simulink model "SafetyChecks"  (R2020b)
settings: Solver=FixedStepDiscrete  StartTime=0.0  StopTime=10.0  FixedStep=4*Ts  RelTol=1e-3
undefined symbols (not defined in the file or in its folder): MaximumCurrentBeforeReaction
libraries: simulink x3
settings Model: DataDictionary=SafetyChecks.sldd  Creator=unix  LastModifiedBy=unix

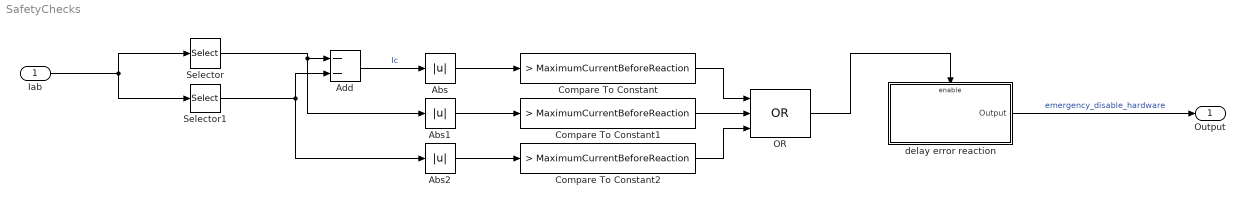
== system SafetyChecks ==
  Iab : Inport  OutDataTypeStr=fixdt(1,16,2^-8,0)
  Abs : Abs
  Abs1 : Abs
  Abs2 : Abs
  Add : Sum  Inputs=--
  Compare To Constant : simulink/Logic and Bit Operations/Compare To Constant  relop=>  const=MaximumCurrentBeforeReaction  OutDataTypeStr=boolean
  Compare To Constant1 : simulink/Logic and Bit Operations/Compare To Constant  relop=>  const=MaximumCurrentBeforeReaction  OutDataTypeStr=boolean
  Compare To Constant2 : simulink/Logic and Bit Operations/Compare To Constant  relop=>  const=MaximumCurrentBeforeReaction  OutDataTypeStr=boolean
  OR : Logic  Operator=OR  Inputs=3  IconShape=distinctive  AllPortsSameDT=off  OutDataTypeStr=boolean
  Selector : Selector  InputPortWidth=2  IndexOptions=Index vector (dialog)  Indices=[1]  OutputSizes=1
  Selector1 : Selector  InputPortWidth=2  IndexOptions=Index vector (dialog)  Indices=[2]  OutputSizes=1
  delay error reaction : Subsystem  TreatAsAtomicUnit=on
  Output : Outport
  wires:
  Iab/1 -> Selector1/1, Selector/1
  Selector/1 -> Abs1/1, Add/1
  Selector1/1 -> Add/2, Abs2/1
  Add/1 -> Abs/1  "Ic"
  Abs2/1 -> Compare To Constant2/1
  Abs1/1 -> Compare To Constant1/1
  Abs/1 -> Compare To Constant/1
  Compare To Constant1/1 -> OR/2
  Compare To Constant/1 -> OR/1
  Compare To Constant2/1 -> OR/3
  delay error reaction/1(Output) -> Output/1  "emergency_disable_hardware"
  OR/1 -> delay error reaction/Enable

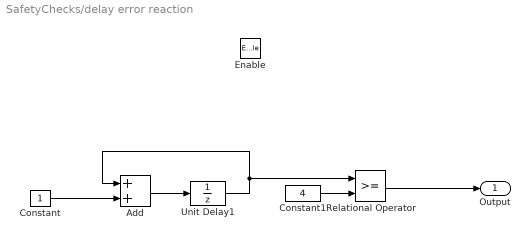
== system SafetyChecks/delay error reaction ==
  Enable : EnablePort  StatesWhenEnabling=reset
  Add : Sum  OutDataTypeStr=uint16
  Constant : Constant  OutDataTypeStr=uint8
  Constant1 : Constant  Value=4  OutDataTypeStr=uint16
  Relational Operator : RelationalOperator  OutDataTypeStr=boolean  RndMeth=Simplest
  Unit Delay1 : UnitDelay  SampleTime=-1  HasFrameUpgradeWarning=on
  Output : Outport  OutputWhenDisabled=reset  InitialOutput=0
      settings: AttributesFormatString=%<InitialOutput>
  wires:
  Add/1 -> Unit Delay1/1
  Unit Delay1/1 -> Relational Operator/1, Add/1
  Constant/1 -> Add/2
  Constant1/1 -> Relational Operator/2
  Relational Operator/1 -> Output/1
